simulink model "doc_fmmoddemod"  (R2016b)
settings: Solver=ode45  StartTime=0.0  StopTime=10  RelTol=1e-3  EnableMultiTasking=on
libraries: commanabbnd3 x2, dspsrcs4 x1
settings Model: Creator=The MathWorks, Inc.  LastModifiedBy=Jawad-PC
settings DataIOCC: LimitDataPoints=on  SaveFormat=Array
settings OptimizationCC: LifeSpan=inf
settings DebuggingCC: SolverPrmCheckMsg=warning  SFUnexpectedBacktrackingDiag=warning  SFNoUnconditionalDefaultTransitionDiag=warning  SFExecutionAtInitializationDiag=none
settings HardwareCC: ProdBitPerPointer=32  ProdBitPerSizeT=32  ProdBitPerPtrDiffT=32  ProdLargestAtomicFloat=None  ProdIntDivRoundTo=Undefined  ProdEndianess=Unspecified  ProdWordSize=32  ProdHWDeviceType=32-bit Generic
settings ModelReferenceCC: PropagateSignalLabelsOutOfModel=off
settings GRTTargetCC: TargetLangStandard=C89/C90 (ANSI)  GeneratePreprocessorConditionals=Disable all
settings ConfigComp: CovMetricSettings=dw  CovHtmlReporting=on  CovSaveCumulativeToWorkspaceVar=on  CovSaveSingleToWorkspaceVar=on  CovExternalEMLEnable=off  CovSFcnEnable=off

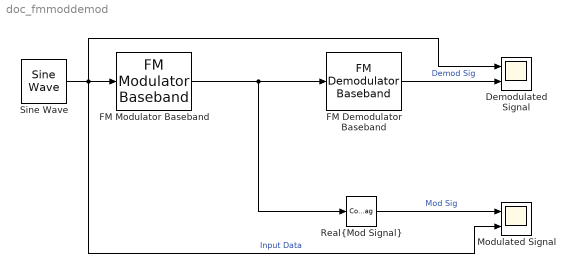
== system doc_fmmoddemod ==
  Demodulated Signal : Scope  NumInputPorts=2
  "FM Demodulator Baseband " : commanabbnd3/FM Demodulator Baseband   FrequencyDeviation=50  SimulateUsing=Interpreted execution
  FM Modulator Baseband : commanabbnd3/FM Modulator Baseband  FrequencyDeviation=50  SimulateUsing=Interpreted execution
  Modulated Signal : Scope  NumInputPorts=2
  "Real{Mod Signal}" : ComplexToRealImag  Output=Real
  Sine Wave : dspsrcs4/Sine Wave  Amplitude=1  Frequency=4  Phase=0  SampleMode=Discrete  OutComplex=Real  CompMethod=Trigonometric fcn  TableSize=Speed  SampleTime=1/1000  SamplesPerFrame=500  ResetState=Restart at time zero  OutputFrames=on  dataType=double  wordLen=16  udDataType=sfix(16)  fracBitsMode=Best precision  numFracBits=15  OutDataTypeStr=double  LastOutDataTypeStr=double
  wires:
  Sine Wave/1 -> Demodulated Signal/1, Modulated Signal/2, FM Modulator Baseband/1  "Input Data"
  FM Modulator Baseband/1 -> "Real{Mod Signal}"/1, "FM Demodulator Baseband "/1
  "Real{Mod Signal}"/1 -> Modulated Signal/1  "Mod Sig"
  "FM Demodulator Baseband "/1 -> Demodulated Signal/2  "Demod Sig"
